simulink model "untitled"  (R2016a)
settings: Solver=FixedStepDiscrete  StartTime=0.0  StopTime=10.0  RelTol=1e-3
settings Model: Creator=SAIC  LastModifiedBy=SAIC

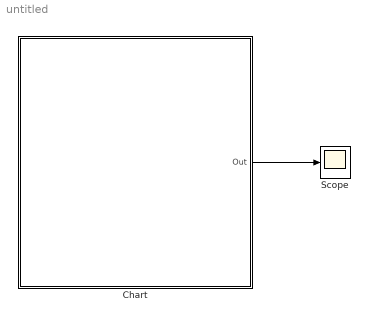
== system untitled ==
  Chart : Stateflow chart  TreatAsAtomicUnit=on
  Scope : Scope
  wires:
  Chart/1(Out) -> Scope/1

== stateflow chart untitled/Chart ==
  state Test
    en:
    Out=0;Counter=0;
    ex:
    Out=1;
    Test -> (junction 5) [order 1]
    (junction 5) -> (junction 9) [order 1] : [Counter<3000]{Counter = Counter + 1}
    (junction 9) -> (junction 5)
    (junction 5) -> (junction 7) [order 2]
  state Test1
  (default) -> Test
  Test -> Test1 [order 1] : [Counter>3000]
  data: Counter local; Out output
